simulink model "lab3_1"  (R2021a)
settings: Solver=VariableStepAuto  StartTime=0.0  StopTime=30  RelTol=10e-10  AbsTol=10e-10
undefined symbols (not defined in the file): a, dbar, K, s, TI, vdes
libraries: cstblocks x2
settings Model: Creator=spencersun  LastModifiedBy=spencersun
settings SolverCC: AlgebraicLoopSolver=TrustRegion
settings DebuggingCC: SFMachineParentedDataDiag=warning

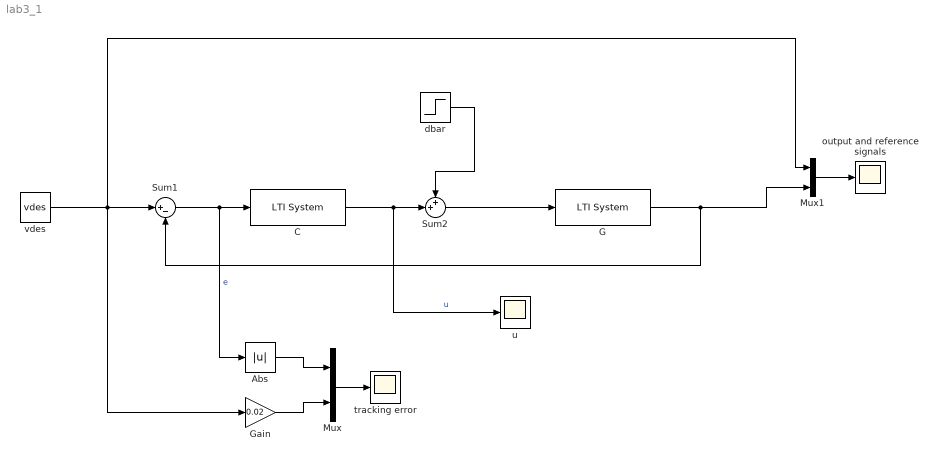
== system lab3_1 ==
  Abs : Abs
  C : cstblocks/LTI System  sys=K*(TI*s + 1)/(TI*s)  IC=[]
  G : cstblocks/LTI System  sys=1/(s+a)  IC=[]
  Gain : Gain  Gain=0.02
  Mux : Mux  Inputs=2
  Mux1 : Mux  Inputs=2
  Sum1 : Sum  Inputs=|+-
  Sum2 : Sum  Inputs=++|
  "dbar " : Step  Time=15  After=dbar  SampleTime=0
  output and reference signals : Scope
  tracking error : Scope
  "u " : Scope
  "vdes " : Constant  Value=vdes
  wires:
  Mux/1 -> tracking error/1
  C/1 -> Sum2/2, "u "/1  "u"
  "dbar "/1 -> Sum2/1
  Sum2/1 -> G/1
  G/1 -> Mux1/2, Sum1/2
  Sum1/1 -> C/1, Abs/1  "e"
  Abs/1 -> Mux/1
  Gain/1 -> Mux/2
  Mux1/1 -> output and reference signals/1
  "vdes "/1 -> Mux1/1, Sum1/1, Gain/1
